simulink model "simulink_problem15"  (R2019b)
settings: Solver=VariableStepAuto  StartTime=0.0  StopTime=2  RelTol=1e-3
values from neighbouring files (symbols this model uses):
  A1 = 1    [problem13.m]    (also in problem15.m = 0.17; problem16.m = 0.17; problem17.m = 0.17; problem18.m = 0.17)
  A2 = 1    [problem13.m]    (also in problem15.m = 0.17; problem16.m = 0.17; problem17.m = 0.17; problem18.m = 0.17)
  A3 = 1    [problem13.m]    (also in problem15.m = 0.17; problem16.m = 0.17; problem17.m = 0.17; problem18.m = 0.17)
  A4 = 1    [problem13.m]    (also in problem15.m = 0.17; problem16.m = 0.17; problem17.m = 0.17; problem18.m = 0.17)
  C1 = n^2 * [J_eff(1)  (f_eff + KT*KD1)  KT*KP1  0]    [problem13.m]    (also in problem15.m = n^2 * d1; problem16.m = n^2 * d1; problem17.m = n^2 * den1; problem18.m = n^2 * den1)
  C2 = n^2 * [J_eff(2)  (f_eff + KT*KD2)  KT*KP2  0]    [problem13.m]    (also in problem15.m = n^2 * d2; problem16.m = n^2 * d2; problem17.m = n^2 * den2; problem18.m = n^2 * den2)
  C3 = n^2 * [J_eff(3)  (f_eff + KT*KD3)  KT*KP3  0]    [problem13.m]    (also in problem15.m = n^2 * d3; problem16.m = n^2 * d3; problem17.m = n^2 * den3; problem18.m = n^2 * den3)
  C4 = n^2 * [J_eff(4)  (f_eff + KT*KD4)  KT*KP4  0]    [problem13.m]    (also in problem15.m = n^2 * d4; problem16.m = n^2 * d4; problem17.m = n^2 * den4; problem18.m = n^2 * den4)
  d1 = [J_eff(1)  (f_eff + KT*KD1)  KT*KP1]    [problem12.m]    (also in problem15.m = [J_eff(1)  (f_eff + KT*KD1)  KT*KP1  KT*KI]; problem16.m = [J_eff(1)  (f_eff + KT*KD1)  KT*KP1  KT*KI]; problem17.m = 1.5; problem18.m = 1.5)
  d2 = [J_eff(2)  (f_eff + KT*KD2)  KT*KP2]    [problem12.m]    (also in problem15.m = [J_eff(2)  (f_eff + KT*KD2)  KT*KP2  KT*KI]; problem16.m = [J_eff(2)  (f_eff + KT*KD2)  KT*KP2  KT*KI])
  d3 = [J_eff(3)  (f_eff + KT*KD3)  KT*KP3]    [problem12.m]    (also in problem15.m = [J_eff(3)  (f_eff + KT*KD3)  KT*KP3  KT*KI]; problem16.m = [J_eff(3)  (f_eff + KT*KD3)  KT*KP3  KT*KI])
  d4 = [J_eff(4)  (f_eff + KT*KD4)  KT*KP4]    [problem12.m]    (also in problem15.m = [J_eff(4)  (f_eff + KT*KD4)  KT*KP4  KT*KI]; problem16.m = [J_eff(4)  (f_eff + KT*KD4)  KT*KP4  KT*KI])
  n1 = KT * [KD1  KP1]    [problem12.m]    (also in problem15.m = KT * [KD1  KP1  KI]; problem16.m = KT * [KD1  KP1  KI])
  n2 = KT * [KD2  KP2]    [problem12.m]    (also in problem15.m = KT * [KD2  KP2  KI]; problem16.m = KT * [KD2  KP2  KI])
  n3 = KT * [KD3  KP3]    [problem12.m]    (also in problem15.m = KT * [KD3  KP3  KI]; problem16.m = KT * [KD3  KP3  KI])
  n4 = KT * [KD4  KP4]    [problem12.m]    (also in problem15.m = KT * [KD4  KP4  KI]; problem16.m = KT * [KD4  KP4  KI])
settings Model: Creator=ben  LastModifiedBy=axeljacobsen

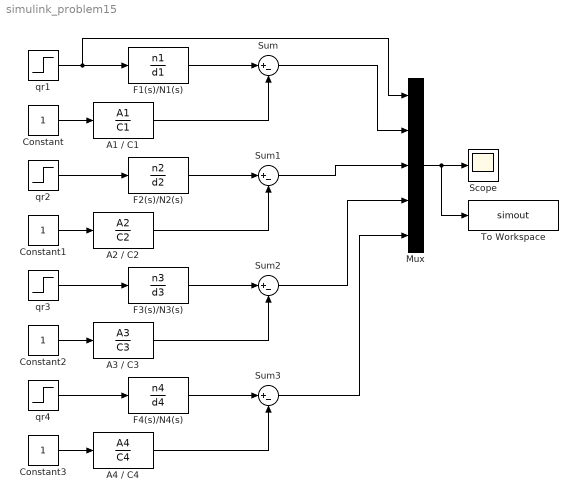
== system simulink_problem15 ==
  A1 / C1 : TransferFcn  Numerator=A1  Denominator=C1
  "A2 / C2 " : TransferFcn  Numerator=A2  Denominator=C2
  "A3 / C3 " : TransferFcn  Numerator=A3  Denominator=C3
  A4 / C4 : TransferFcn  Numerator=A4  Denominator=C4
  Constant{,1..3} (4 alike) : Constant
  F1(s)/N1(s) : TransferFcn  Numerator=n1  Denominator=d1
  F2(s)/N2(s) : TransferFcn  Numerator=n2  Denominator=d2
  F3(s)/N3(s) : TransferFcn  Numerator=n3  Denominator=d3
  F4(s)/N4(s) : TransferFcn  Numerator=n4  Denominator=d4
  Mux : Mux  Inputs=5
  Scope : Scope
  Sum{,1..3} (4 alike) : Sum  Inputs=|+-
  To Workspace : ToWorkspace  VariableName=simout  SampleTime=-1
  qr{1..4} (4 alike) : Step  Time=0.5  After=0.35  SampleTime=0
  wires:
  qr1/1 -> Mux/1, F1(s)/N1(s)/1
  Mux/1 -> To Workspace/1, Scope/1
  qr4/1 -> F4(s)/N4(s)/1
  qr2/1 -> F2(s)/N2(s)/1
  qr3/1 -> F3(s)/N3(s)/1
  F1(s)/N1(s)/1 -> Sum/1
  Sum/1 -> Mux/2
  A1 / C1/1 -> Sum/2
  Sum1/1 -> Mux/3
  "A2 / C2 "/1 -> Sum1/2
  F2(s)/N2(s)/1 -> Sum1/1
  Sum2/1 -> Mux/4
  F3(s)/N3(s)/1 -> Sum2/1
  "A3 / C3 "/1 -> Sum2/2
  Sum3/1 -> Mux/5
  F4(s)/N4(s)/1 -> Sum3/1
  A4 / C4/1 -> Sum3/2
  Constant/1 -> A1 / C1/1
  Constant1/1 -> "A2 / C2 "/1
  Constant2/1 -> "A3 / C3 "/1
  Constant3/1 -> A4 / C4/1
